simulink model "Observador_Seguidor_Integradores"  (R2016a)
settings: Solver=VariableStepAuto  StartTime=0.0  StopTime=550  RelTol=1e-3
undefined symbols (not defined in the file): A, B, C, K, Ki, Kx, L
settings Model: Creator=Caeta  LastModifiedBy=Caeta

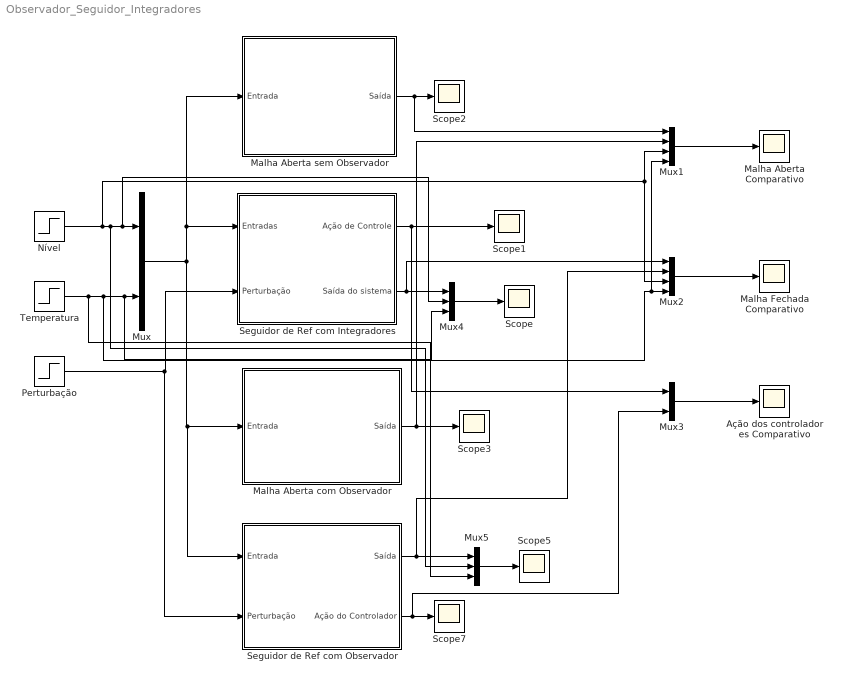
== system Observador_Seguidor_Integradores ==
  Ação dos controladores Comparativo : Scope
  Malha Aberta Comparativo : Scope
  Malha Aberta com Observador : Subsystem
  Malha Aberta sem Observador : Subsystem
  Malha Fechada Comparativo : Scope
  Mux : Mux  Inputs=2
  Mux1 : Mux
  Mux2 : Mux
  Mux3 : Mux  Inputs=2
  Mux4 : Mux  Inputs=3
  Mux5 : Mux  Inputs=3
  Nível : Step  SampleTime=0
  Perturbação : Step  Time=350  SampleTime=0
  Scope{,1..3,5,7} (6 alike) : Scope
  Seguidor de Ref com Integradores : Subsystem
  Seguidor de Ref com Observador : Subsystem
  Temperatura : Step  Time=250  SampleTime=0
  wires:
  Temperatura/1 -> Mux5/3, Mux1/4, Mux2/4, Mux4/3, Mux/2
  Seguidor de Ref com Integradores/1(Ação de Controle) -> Scope1/1, Mux3/1
  Seguidor de Ref com Integradores/2(Saída do sistema) -> Mux4/1, Mux2/1
  Malha Aberta sem Observador/1(Saída) -> Scope2/1, Mux1/1
  Mux/1 -> Seguidor de Ref com Integradores/1(Entradas), Malha Aberta sem Observador/1(Entrada), Seguidor de Ref com Observador/1(Entrada), Malha Aberta com Observador/1(Entrada)
  Malha Aberta com Observador/1(Saída) -> Mux1/2, Scope3/1
  Seguidor de Ref com Observador/2(Ação do Controlador) -> Mux3/2, Scope7/1
  Mux1/1 -> Malha Aberta Comparativo/1
  Seguidor de Ref com Observador/1(Saída) -> Mux5/1, Mux2/2
  Mux2/1 -> Malha Fechada Comparativo/1
  Mux3/1 -> Ação dos controladores Comparativo/1
  Nível/1 -> Mux1/3, Mux2/3, Mux5/2, Mux4/2, Mux/1
  Perturbação/1 -> Seguidor de Ref com Observador/2(Perturbação), Seguidor de Ref com Integradores/2(Perturbação)
  Mux5/1 -> Scope5/1
  Mux4/1 -> Scope/1

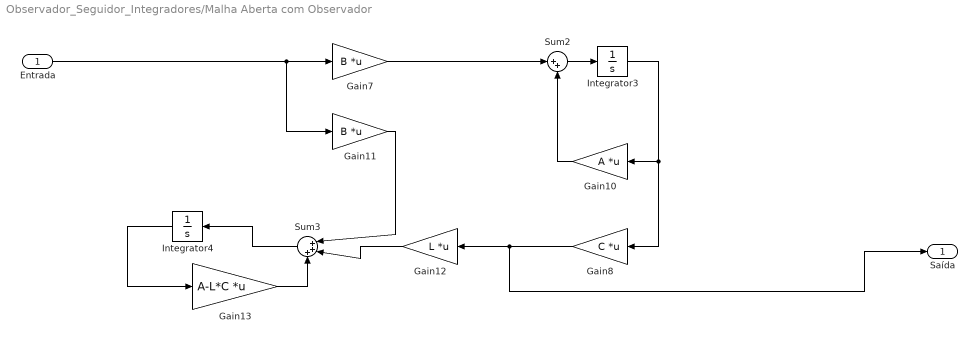
== system Observador_Seguidor_Integradores/Malha Aberta com Observador ==
  Entrada : Inport
  Gain10 : Gain  Gain=A  Multiplication=Matrix(K*u)
  Gain11 : Gain  Gain=B  Multiplication=Matrix(K*u)
  Gain12 : Gain  Gain=L  Multiplication=Matrix(K*u)
  Gain13 : Gain  Gain=A-L*C  Multiplication=Matrix(K*u)
  Gain7 : Gain  Gain=B  Multiplication=Matrix(K*u)
  Gain8 : Gain  Gain=C  Multiplication=Matrix(K*u)
  Integrator3 : Integrator
  Integrator4 : Integrator
  Sum2 : Sum  Inputs=|++
  Sum3 : Sum  Inputs=|+++
  Saída : Outport
  wires:
  Gain10/1 -> Sum2/2
  Sum3/1 -> Integrator4/1
  Gain8/1 -> Saída/1, Gain12/1
  Sum2/1 -> Integrator3/1
  Integrator3/1 -> Gain8/1, Gain10/1
  Entrada/1 -> Gain11/1, Gain7/1
  Gain11/1 -> Sum3/1
  Gain13/1 -> Sum3/3
  Integrator4/1 -> Gain13/1
  Gain7/1 -> Sum2/1
  Gain12/1 -> Sum3/2

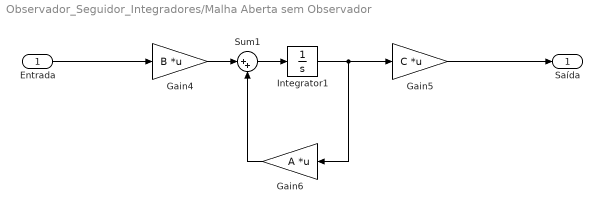
== system Observador_Seguidor_Integradores/Malha Aberta sem Observador ==
  Entrada : Inport
  Gain4 : Gain  Gain=B  Multiplication=Matrix(K*u)
  Gain5 : Gain  Gain=C  Multiplication=Matrix(K*u)
  Gain6 : Gain  Gain=A  Multiplication=Matrix(K*u)
  Integrator1 : Integrator
  Sum1 : Sum  Inputs=|++
  Saída : Outport
  wires:
  Gain4/1 -> Sum1/1
  Gain6/1 -> Sum1/2
  Sum1/1 -> Integrator1/1
  Integrator1/1 -> Gain5/1, Gain6/1
  Gain5/1 -> Saída/1
  Entrada/1 -> Gain4/1

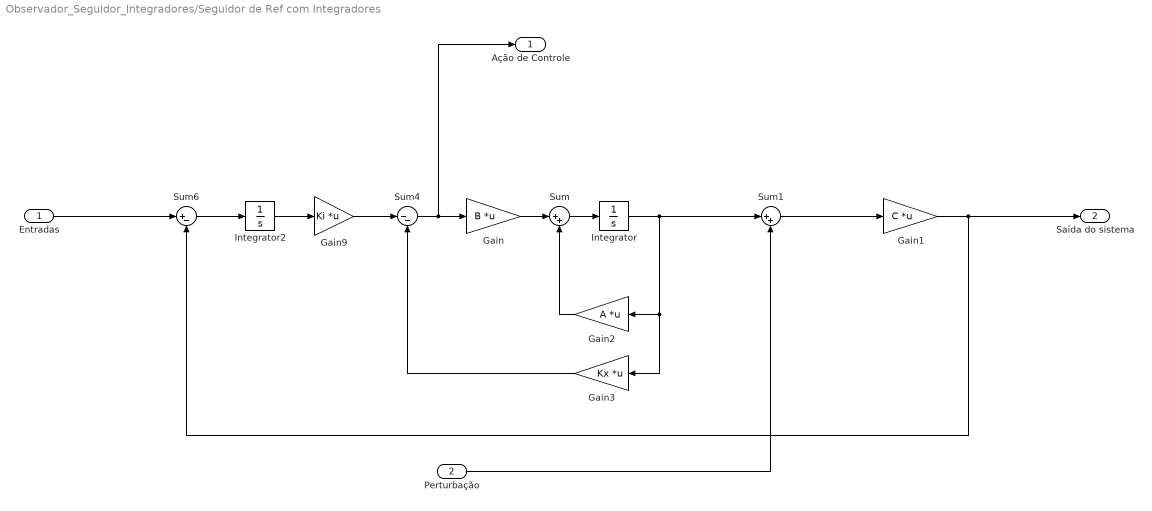
== system Observador_Seguidor_Integradores/Seguidor de Ref com Integradores ==
  Entradas : Inport
  Perturbação : Inport  Port=2
  Gain : Gain  Gain=B  Multiplication=Matrix(K*u)
  Gain1 : Gain  Gain=C  Multiplication=Matrix(K*u)
  Gain2 : Gain  Gain=A  Multiplication=Matrix(K*u)
  Gain3 : Gain  Gain=Kx  Multiplication=Matrix(K*u)
  Gain9 : Gain  Gain=Ki  Multiplication=Matrix(K*u)
  Integrator : Integrator
  Integrator2 : Integrator
  Sum : Sum  Inputs=|++
  Sum1 : Sum  Inputs=|++
  Sum4 : Sum  Inputs=|--
  Sum6 : Sum  Inputs=|+-
  Ação de Controle : Outport
  Saída do sistema : Outport  Port=2
  wires:
  Integrator2/1 -> Gain9/1
  Gain9/1 -> Sum4/1
  Entradas/1 -> Sum6/1
  Sum/1 -> Integrator/1
  Sum4/1 -> Ação de Controle/1, Gain/1
  Sum6/1 -> Integrator2/1
  Integrator/1 -> Sum1/1, Gain3/1, Gain2/1
  Gain3/1 -> Sum4/2
  Gain2/1 -> Sum/2
  Gain/1 -> Sum/1
  Gain1/1 -> Saída do sistema/1, Sum6/2
  Sum1/1 -> Gain1/1
  Perturbação/1 -> Sum1/2

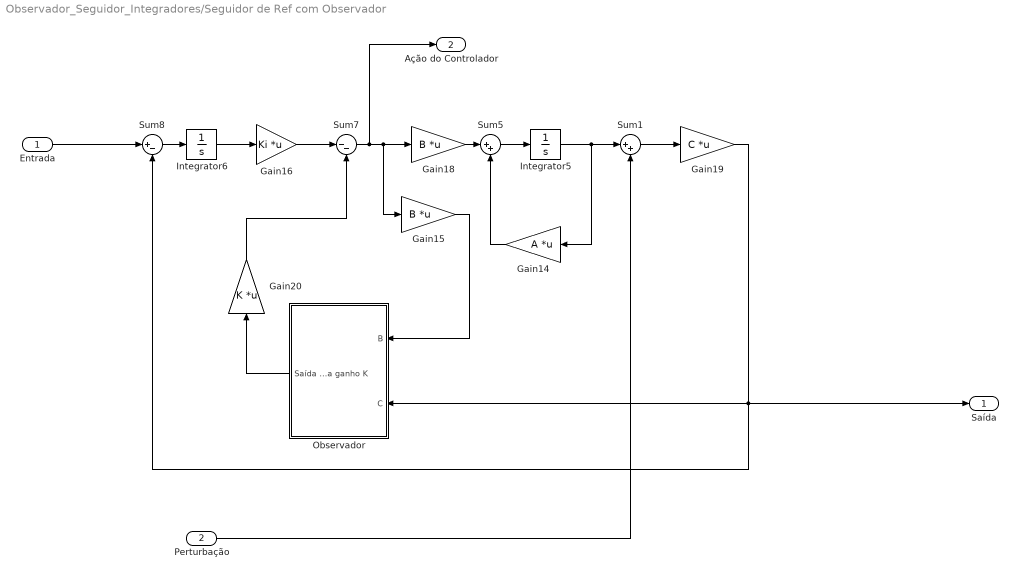
== system Observador_Seguidor_Integradores/Seguidor de Ref com Observador ==
  Entrada : Inport
  Perturbação : Inport  Port=2
  Gain14 : Gain  Gain=A  Multiplication=Matrix(K*u)
  Gain15 : Gain  Gain=B  Multiplication=Matrix(K*u)
  Gain16 : Gain  Gain=Ki  Multiplication=Matrix(K*u)
  Gain18 : Gain  Gain=B  Multiplication=Matrix(K*u)
  Gain19 : Gain  Gain=C  Multiplication=Matrix(K*u)
  Gain20 : Gain  Gain=K  Multiplication=Matrix(K*u)
  Integrator5 : Integrator
  Integrator6 : Integrator
  Observador : Subsystem
  Sum1 : Sum  Inputs=|++
  Sum5 : Sum  Inputs=|++
  Sum7 : Sum  Inputs=|--
  Sum8 : Sum  Inputs=|+-
  Saída : Outport
  Ação do Controlador : Outport  Port=2
  wires:
  Gain20/1 -> Sum7/2
  Gain15/1 -> Observador/1(B)
  Observador/1(Saída para ganho K) -> Gain20/1
  Integrator5/1 -> Sum1/1, Gain14/1
  Sum5/1 -> Integrator5/1
  Gain14/1 -> Sum5/2
  Gain18/1 -> Sum5/1
  Entrada/1 -> Sum8/1
  Gain16/1 -> Sum7/1
  Sum7/1 -> Ação do Controlador/1, Gain15/1, Gain18/1
  Integrator6/1 -> Gain16/1
  Sum8/1 -> Integrator6/1
  Sum1/1 -> Gain19/1
  Perturbação/1 -> Sum1/2
  Gain19/1 -> Observador/2(C), Sum8/2, Saída/1

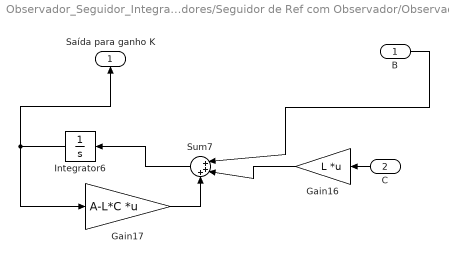
== system Observador_Seguidor_Integradores/Seguidor de Ref com Observador/Observador ==
  B : Inport
  C : Inport  Port=2
  Gain16 : Gain  Gain=L  Multiplication=Matrix(K*u)
  Gain17 : Gain  Gain=A-L*C  Multiplication=Matrix(K*u)
  Integrator6 : Integrator
  Sum7 : Sum  Inputs=|+++
  Saída para ganho K : Outport
  wires:
  C/1 -> Gain16/1
  Gain17/1 -> Sum7/3
  Sum7/1 -> Integrator6/1
  Integrator6/1 -> Saída para ganho K/1, Gain17/1
  B/1 -> Sum7/1
  Gain16/1 -> Sum7/2
